simulink model "Model_aircraft_simple_fly"  (R2024b)
settings: Solver=VariableStepAuto  StartTime=0.0  StopTime=T_fin  RelTol=1e-3
settings Model: Creator=dragom  LastModifiedBy=gregor
settings RTWCC: GPUComputeCapability=3.5

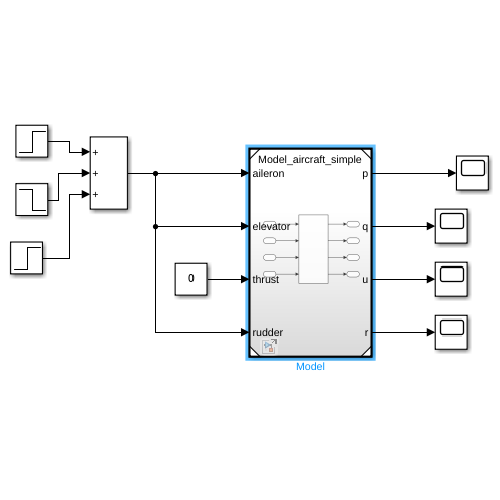
[thumbnail: Simulink's stored preview of the top-level diagram]
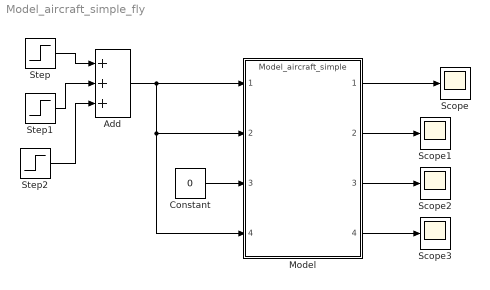
== system Model_aircraft_simple_fly ==
  Add : Sum  Inputs=+++
  Constant : Constant  Value=0
  Model : ModelReference  ModelNameDialog=Model_aircraft_simple.slx  SimulationMode=Normal  ModelReferenceVersion=21.1
  Scope{,1..3} (4 alike) : Scope
  Step : Step  Time=10  SampleTime=0
  Step1 : Step  Time=11  After=-2  SampleTime=0
  Step2 : Step  Time=12  SampleTime=0
  wires:
  Step2/1 -> Add/3
  Step1/1 -> Add/2
  Step/1 -> Add/1
  Constant/1 -> Model/3
  Model/1 -> Scope/1
  Model/2 -> Scope1/1
  Model/3 -> Scope2/1
  Model/4 -> Scope3/1
  Add/1 -> Model/4, Model/2, Model/1
